simulink model "lab1"  (R2020b)
settings: Solver=VariableStepAuto  StartTime=0.0  StopTime=10.0  RelTol=1e-3
settings Model: Creator=BIDITA PAUL  LastModifiedBy=BIDITA PAUL

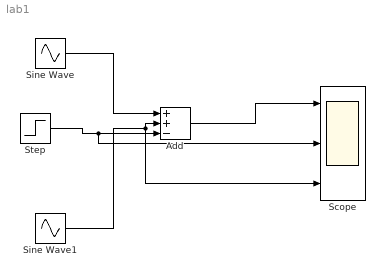
== system lab1 ==
  Add : Sum  Inputs=++-
  Scope : Scope  NumInputPorts=3
  Sine Wave : Sin  SampleTime=0
  Sine Wave1 : Sin  Frequency=4  SampleTime=0
  Step : Step  SampleTime=0
  wires:
  Sine Wave/1 -> Add/1
  Sine Wave1/1 -> Scope/3, Add/2
  Add/1 -> Scope/1
  Step/1 -> Scope/2, Add/3
